simulink model "sys"  (R2017a)
settings: Solver=VariableStepAuto  StartTime=0.0  StopTime=40  FixedStep=0.02  RelTol=1e-3
values from neighbouring files (symbols this model uses):
  D = zeros(1,1)    [OBS_CONT.m]
  F = [0 1 0 0;-k/j2 -b/j2 k/j2 b/j2;0 0 0 01;k/j1 b/j1 -k/j1 -b/j1]    [OBS_CONT.m]
  G = [0;0;0;1/j1]    [OBS_CONT.m]
  H = [1 0 0 0]    [OBS_CONT.m]
  Kc = [-0.26139 0.041515 0.65538 1.1604]    [OBS_CONT.m]    (also in OBS_CONT_MORE_STIFF.m = place(F,G,p_cont))
  Ke = [22.0004 242.0531 1512.84032 5485.9822]'    [OBS_CONT.m]    (also in OBS_CONT_MORE_STIFF.m = Ke')
  Kr = rscale(F,G,H,D,Kc)    [OBS_CONT.m]    (also in OBS_CONT_MORE_STIFF.m)
settings Model: Creator=ASUS  LastModifiedBy=ASUS

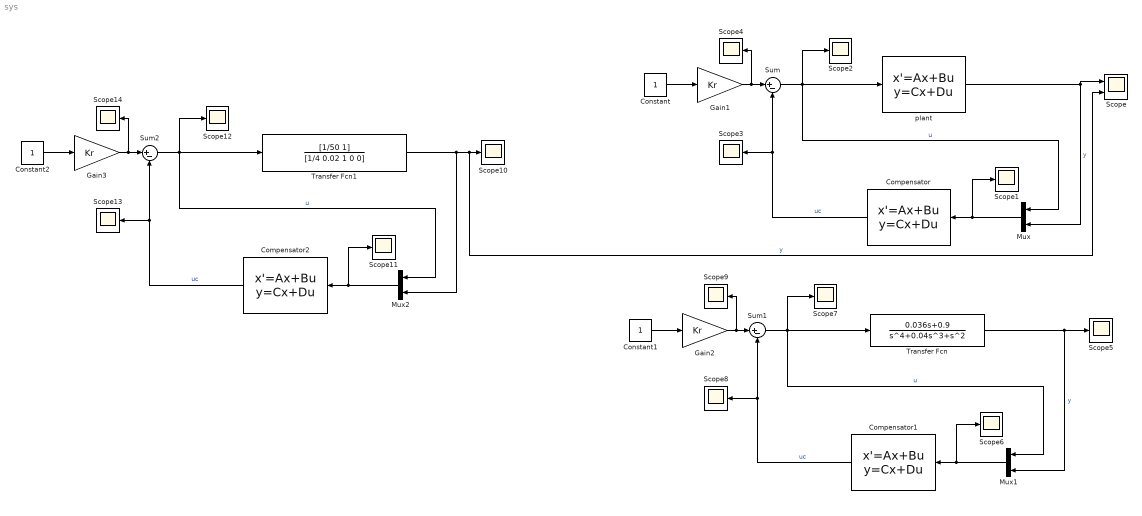
== system sys ==
  Compensator : StateSpace  A=F-Ke*H  B=[G Ke]  C=Kc  D=[D D]  X0=0
  Compensator1 : StateSpace  A=F-Ke*H  B=[G Ke]  C=Kc  D=[D D]  X0=0
  Compensator2 : StateSpace  A=F-Ke*H  B=[G Ke]  C=Kc  D=[D D]  X0=0
  Constant : Constant
  Constant1 : Constant
  Constant2 : Constant
  Gain1 : Gain  Gain=Kr
  Gain2 : Gain  Gain=Kr
  Gain3 : Gain  Gain=Kr
  Mux : Mux  Inputs=2
  Mux1 : Mux  Inputs=2
  Mux2 : Mux  Inputs=2
  Scope : Scope  NumInputPorts=2
  Scope{1..14} (14 alike) : Scope
  Sum : Sum  Inputs=|+-
  Sum1 : Sum  Inputs=|+-
  Sum2 : Sum  Inputs=|+-
  Transfer Fcn : TransferFcn  Numerator=[0.036 0.9]  Denominator=[1 0.04 1 0 0]
  Transfer Fcn1 : TransferFcn  Numerator=[1/50 1]  Denominator=[1/4 0.02 1 0 0]
  plant : StateSpace  A=F  B=G  C=H  D=D  X0=0
  wires:
  Sum/1 -> Scope2/1, Mux/1, plant/1  "u"
  plant/1 -> Mux/2, Scope/1  "y"
  Compensator/1 -> Scope3/1, Sum/2  "uc"
  Constant/1 -> Gain1/1
  Gain1/1 -> Scope4/1, Sum/1
  Mux/1 -> Scope1/1, Compensator/1
  Mux1/1 -> Compensator1/1, Scope6/1
  Gain2/1 -> Sum1/1, Scope9/1
  Constant1/1 -> Gain2/1
  Compensator1/1 -> Sum1/2, Scope8/1  "uc"
  Transfer Fcn/1 -> Scope5/1, Mux1/2  "y"
  Sum1/1 -> Transfer Fcn/1, Mux1/1, Scope7/1  "u"
  Transfer Fcn1/1 -> Scope10/1, Scope/2, Mux2/2  "y"
  Sum2/1 -> Transfer Fcn1/1, Mux2/1, Scope12/1  "u"
  Compensator2/1 -> Sum2/2, Scope13/1  "uc"
  Mux2/1 -> Compensator2/1, Scope11/1
  Gain3/1 -> Sum2/1, Scope14/1
  Constant2/1 -> Gain3/1
